simulink library "wt_blockset_beta"  (Simulink 5.0)
values from neighbouring files (symbols this model uses):
  a = -Le\Re    [matrix_coeff_trafo3limb_abc.m]
  a11 = K2*Rs/Ls    [matrix_coeff_scim_abc.m]    (also in matrix_coeff_spsm_dq.m = -Rs*Ksgm_frd/Ksgm_d; matrix_coeff_trafo_abc.m = K2*Rhv/Lhv; matrix_coeff_wrim_abc.m)
  a12 = K3*Rs/Ls    [matrix_coeff_scim_abc.m]    (also in matrix_coeff_spsm_dq.m = Lssq*Ksgm_frd/Ksgm_d; matrix_coeff_trafo_abc.m = K3*Rhv/Lhv; matrix_coeff_wrim_abc.m)
  a13 = 3*Msr*sqrt(3)*K4/4    [matrix_coeff_scim_abc.m]    (also in matrix_coeff_spsm_dq.m = Rf*Lsgm_rd*Lmd/Ksgm_d; matrix_coeff_trafo_abc.m = K4*Rhv; matrix_coeff_wrim_abc.m)
  a14 = K4*Rr    [matrix_coeff_scim_abc.m]    (also in matrix_coeff_spsm_dq.m = Rrd*Lsgm_f*Lmd/Ksgm_d; matrix_coeff_trafo_abc.m = K2/Lhv; matrix_coeff_wrim_abc.m)
  a15 = Msr*(K2-K3)/Ls    [matrix_coeff_scim_abc.m]    (also in matrix_coeff_spsm_dq.m = Lmq*Ksgm_frd/Ksgm_d; matrix_coeff_trafo_abc.m = K3/Lhv; matrix_coeff_wrim_abc.m)
  a16 = K2/Ls    [matrix_coeff_scim_abc.m]    (also in matrix_coeff_spsm_dq.m = Ksgm_frd/Ksgm_d; matrix_coeff_trafo_abc.m = K4; matrix_coeff_wrim_abc.m)
  a17 = K3/Ls    [matrix_coeff_scim_abc.m]    (also in matrix_coeff_spsm_dq.m = -Lsgm_rd*Lmd/Ksgm_d; matrix_coeff_wrim_abc.m)
  a21 = -Lssd*Lsrq/Ksgm_q    [matrix_coeff_spsm_dq.m]
  a22 = -Rs*Lsrq/Ksgm_q    [matrix_coeff_spsm_dq.m]
  a23 = -Lsrq*Lmd/Ksgm_q    [matrix_coeff_spsm_dq.m]
  a24 = -Lsrq*Lmd/Ksgm_q    [matrix_coeff_spsm_dq.m]
  a25 = Rrq*Lmq/Ksgm_q    [matrix_coeff_spsm_dq.m]
  a26 = Lsrq/Ksgm_q    [matrix_coeff_spsm_dq.m]
  a31 = K4*Rs    [matrix_coeff_scim_abc.m]    (also in matrix_coeff_spsm_dq.m = +Rs*Lsgm_rd*Lmd/Ksgm_d; matrix_coeff_trafo_abc.m = K4*Rlv; matrix_coeff_wrim_abc.m)
  a32 = Msr*(K2-K3)/Lr    [matrix_coeff_scim_abc.m]    (also in matrix_coeff_spsm_dq.m = -Lssq*Lsgm_rd*Lmd/Ksgm_d; matrix_coeff_trafo_abc.m = K2*Rlv/Llv; matrix_coeff_wrim_abc.m)
  a33 = K2*Rr/Lr    [matrix_coeff_scim_abc.m]    (also in matrix_coeff_spsm_dq.m = -Rf*Ksgm_srd/Ksgm_d; matrix_coeff_trafo_abc.m = K3*Rlv/Llv; matrix_coeff_wrim_abc.m)
  a34 = K3*Rr/Lr    [matrix_coeff_scim_abc.m]    (also in matrix_coeff_spsm_dq.m = Rrd*Lsgm_s*Lmd/Ksgm_d; matrix_coeff_trafo_abc.m = K4; matrix_coeff_wrim_abc.m)
  a35 = 3*Msr*sqrt(3)*K4/4    [matrix_coeff_scim_abc.m]    (also in matrix_coeff_spsm_dq.m = -Lsgm_rd*Lmd*Lmq/Ksgm_d; matrix_coeff_trafo_abc.m = K2/Llv; matrix_coeff_wrim_abc.m)
  a36 = K4    [matrix_coeff_scim_abc.m]    (also in matrix_coeff_spsm_dq.m = -Lsgm_rd*Lmd/Ksgm_d; matrix_coeff_trafo_abc.m = K3/Llv; matrix_coeff_wrim_abc.m)
  a37 = Ksgm_srd/Ksgm_d    [matrix_coeff_spsm_dq.m]    (also in matrix_coeff_wrim_abc.m = K2/Lr)
  a41 = Rs*Lsgm_f*Lmd/Ksgm_d    [matrix_coeff_spsm_dq.m]
  a42 = -Lsgm_f*Lssq*Lmd/Ksgm_d    [matrix_coeff_spsm_dq.m]
  a43 = Rf*Lsgm_s*Lmd/Ksgm_d    [matrix_coeff_spsm_dq.m]
  a44 = -Rrd*Ksgm_sf/Ksgm_d    [matrix_coeff_spsm_dq.m]
  a45 = -Lsgm_f*Lmd*Lmq/Ksgm_d    [matrix_coeff_spsm_dq.m]
  a46 = -Lsgm_f*Lmd/Ksgm_d    [matrix_coeff_spsm_dq.m]
  a47 = -Lsgm_s*Lmd/Ksgm_d    [matrix_coeff_spsm_dq.m]
  a51 = Lssd*Lmq/Ksgm_q    [matrix_coeff_spsm_dq.m]
  a52 = Rs*Lmq/Ksgm_q    [matrix_coeff_spsm_dq.m]
  a53 = Lmd*Lmq/Ksgm_q    [matrix_coeff_spsm_dq.m]
  a54 = Lmd*Lmq/Ksgm_q    [matrix_coeff_spsm_dq.m]
  a55 = -Rrq*Lssq/Ksgm_q    [matrix_coeff_spsm_dq.m]
  a56 = -Lmq/Ksgm_q    [matrix_coeff_spsm_dq.m]
  alpha_T = Ubase_hv/Ubase_lv    [matrix_coeff_trafo3limb_abc.m]
  b = inv(Le)    [matrix_coeff_trafo3limb_abc.m]
  Ctorque = cq(2:5:102,2:5:182)    [cq_table.m]
  Lmd = mag_ind(1)    [matrix_coeff_spsm_dq.m]
  Lmq = mag_ind(2)    [matrix_coeff_spsm_dq.m]
  Lss = Lsgms+Lm    [init_dbe_dq_scim.m]
  omg_base = 2*pi*rated_fp(1)    [init_dbe_dq_scim.m]    (also in init_dbe_rms_scim.m)
  p = rated_fp(2)    [init_dbe_dq_scim.m]    (also in init_dbe_rms_scim.m)
  Rs = stator(1)    [init_dbe_dq_scim.m]    (also in init_dbe_rms_scim.m; matrix_coeff_scim_abc.m; matrix_coeff_spsm_dq.m = stator_winding(1); matrix_coeff_wrim_abc.m)
  Xs = omg_base*Lss    [init_dbe_dq_scim.m]    (also in init_dbe_rms_scim.m = Xsgm_s+Xm)
undefined symbols (not defined in the file or in its folder): get, j, Kmode, ModeOp, Type, u0
libraries: simulink_extras x12, simulink x4, dspinverses x1, dspmtrx3 x1, dspsigattribs x1, dspspect3 x1
(part 4 of 4)

== system wt_blockset_beta/Mechanical Components/Wind Model SB-2/Kaimal_Filter_2/Kaimal Filter ==
  avg_wind : Inport
  In : Inport  Port=2
  A/D : Gain  Gain=0.0182/1.3463  SaturateOnIntegerOverflow=on
  Coefficients : Subsystem
  Integrator : Integrator  Orientation=up
  Integrator1 : Integrator  Orientation=up
  Product : Product  SaturateOnIntegerOverflow=on
  Product1 : Product  SaturateOnIntegerOverflow=on
  Product2 : Product  Orientation=left  SaturateOnIntegerOverflow=on
  Product3 : Product  Orientation=left  SaturateOnIntegerOverflow=on
  Sum : Sum  Inputs=|++  SaturateOnIntegerOverflow=on
  Sum1 : Sum  Orientation=up  Inputs=++-  SaturateOnIntegerOverflow=on
  Sum2 : Sum  Orientation=up  Inputs=+|-  SaturateOnIntegerOverflow=on
  Out : Outport
  wires:
  avg_wind/1 -> Coefficients/1(avg_wind)
  Coefficients/4(FD) -> [FD]
  Coefficients/3(ED) -> [ED]
  Coefficients/2(CD) -> [CD]
  Coefficients/1(BD) -> [BD]
  [FD] -> Product3/2
  [ED] -> Product2/2
  [CD] -> Product1/2
  [BD] -> Product/2
  In/1 -> Product1/1, Product/1, A/D/1
  Sum/1 -> Out/1, Product3/1, Product2/1
  Product1/1 -> Sum2/1
  Product3/1 -> Sum2/2
  Sum2/1 -> Integrator1/1
  Product2/1 -> Sum1/3
  Integrator1/1 -> Sum1/2
  Product/1 -> Sum1/1
  Sum1/1 -> Integrator/1
  Integrator/1 -> Sum/2
  A/D/1 -> Sum/1

== system wt_blockset_beta/Mechanical Components/Wind Model SB-2/Kaimal_Filter_3/Kaimal Filter ==
  avg_wind : Inport
  In : Inport  Port=2
  A/D : Gain  Gain=0.0182/1.3463  SaturateOnIntegerOverflow=on
  Coefficients : Subsystem
  Integrator : Integrator  Orientation=up
  Integrator1 : Integrator  Orientation=up
  Product : Product  SaturateOnIntegerOverflow=on
  Product1 : Product  SaturateOnIntegerOverflow=on
  Product2 : Product  Orientation=left  SaturateOnIntegerOverflow=on
  Product3 : Product  Orientation=left  SaturateOnIntegerOverflow=on
  Sum : Sum  Inputs=|++  SaturateOnIntegerOverflow=on
  Sum1 : Sum  Orientation=up  Inputs=++-  SaturateOnIntegerOverflow=on
  Sum2 : Sum  Orientation=up  Inputs=+|-  SaturateOnIntegerOverflow=on
  Out : Outport
  wires:
  A/D/1 -> Sum/1
  Integrator/1 -> Sum/2
  Sum1/1 -> Integrator/1
  Product/1 -> Sum1/1
  Integrator1/1 -> Sum1/2
  Product2/1 -> Sum1/3
  Sum2/1 -> Integrator1/1
  Product3/1 -> Sum2/2
  Product1/1 -> Sum2/1
  Sum/1 -> Product2/1, Product3/1, Out/1
  In/1 -> A/D/1, Product/1, Product1/1
  [BD] -> Product/2
  [CD] -> Product1/2
  [ED] -> Product2/2
  [FD] -> Product3/2
  Coefficients/1(BD) -> [BD]
  Coefficients/2(CD) -> [CD]
  Coefficients/3(ED) -> [ED]
  Coefficients/4(FD) -> [FD]
  avg_wind/1 -> Coefficients/1(avg_wind)

== system wt_blockset_beta/Mechanical Components/Wind Model SB-2/ZERO_Harmonic_Filter/ZERO harmonic Filter ==
  avg_wind : Inport
  In : Inport  Port=2
  Coefficients : Subsystem
  Integrator : Integrator  Orientation=up
  Integrator1 : Integrator  Orientation=up
  Product : Product  SaturateOnIntegerOverflow=on
  Product1 : Product  SaturateOnIntegerOverflow=on
  Product2 : Product  Orientation=left  SaturateOnIntegerOverflow=on
  Product3 : Product  Orientation=left  SaturateOnIntegerOverflow=on
  Sum1 : Sum  Orientation=up  Inputs=++-  SaturateOnIntegerOverflow=on
  Sum2 : Sum  Orientation=up  Inputs=+|-  SaturateOnIntegerOverflow=on
  Out : Outport
  wires:
  avg_wind/1 -> Coefficients/1(avg_wind)
  Coefficients/4(FD) -> [FD]
  Coefficients/3(ED) -> [ED]
  Coefficients/2(CD) -> [CD]
  Coefficients/1(BD) -> [BD]
  [FD] -> Product3/2
  [ED] -> Product2/2
  [CD] -> Product1/2
  [BD] -> Product/2
  In/1 -> Product1/1, Product/1
  Product1/1 -> Sum2/1
  Product3/1 -> Sum2/2
  Sum2/1 -> Integrator1/1
  Product2/1 -> Sum1/3
  Integrator1/1 -> Sum1/2
  Product/1 -> Sum1/1
  Sum1/1 -> Integrator/1
  Integrator/1 -> Out/1, Product3/1, Product2/1

== system wt_blockset_beta/Power Converters/3-phase Diode Bridge Rectifier/Diode  State Calculator/Branch A+ ==
  RST : Inport
  Demux2 : Demux  Outputs=3
  Logical Operator : Logic
  Relational Operator : RelationalOperator  InputSameDT=on
  Relational Operator1 : RelationalOperator  Operator=>  InputSameDT=on
  A : Outport  InitialOutput=0
  wires:
  Relational Operator/1 -> Logical Operator/1
  Relational Operator1/1 -> Logical Operator/2
  Logical Operator/1 -> A/1
  RST/1 -> Demux2/1
  Demux2/1 -> Relational Operator/1, Relational Operator1/1
  Demux2/3 -> Relational Operator/2
  Demux2/2 -> Relational Operator1/2

== system wt_blockset_beta/Power Converters/3-phase Diode Bridge Rectifier/Diode  State Calculator/Branch A- ==
  RST : Inport
  Demux2 : Demux  Outputs=3
  Logical Operator : Logic
  Relational Operator : RelationalOperator  Operator=<  InputSameDT=on
  Relational Operator1 : RelationalOperator  Operator=<  InputSameDT=on
  A : Outport  InitialOutput=0
  wires:
  Demux2/2 -> Relational Operator1/2
  Demux2/3 -> Relational Operator/2
  Demux2/1 -> Relational Operator1/1, Relational Operator/1
  RST/1 -> Demux2/1
  Logical Operator/1 -> A/1
  Relational Operator1/1 -> Logical Operator/2
  Relational Operator/1 -> Logical Operator/1

== system wt_blockset_beta/Power Converters/3-phase Diode Bridge Rectifier/Diode  State Calculator/Branch B+ ==
  RST : Inport
  Demux2 : Demux  Outputs=3
  Logical Operator : Logic
  Relational Operator : RelationalOperator  InputSameDT=on
  Relational Operator1 : RelationalOperator  Operator=>  InputSameDT=on
  B : Outport  InitialOutput=0
  wires:
  RST/1 -> Demux2/1
  Logical Operator/1 -> B/1
  Relational Operator1/1 -> Logical Operator/2
  Relational Operator/1 -> Logical Operator/1
  Demux2/2 -> Relational Operator/1, Relational Operator1/1
  Demux2/1 -> Relational Operator/2
  Demux2/3 -> Relational Operator1/2

== system wt_blockset_beta/Power Converters/3-phase Diode Bridge Rectifier/Diode  State Calculator/Branch B- ==
  RST : Inport
  Demux2 : Demux  Outputs=3
  Logical Operator : Logic
  Relational Operator : RelationalOperator  Operator=<  InputSameDT=on
  Relational Operator1 : RelationalOperator  Operator=<  InputSameDT=on
  B : Outport  InitialOutput=0
  wires:
  Demux2/3 -> Relational Operator1/2
  Demux2/1 -> Relational Operator/2
  Demux2/2 -> Relational Operator1/1, Relational Operator/1
  Relational Operator/1 -> Logical Operator/1
  Relational Operator1/1 -> Logical Operator/2
  Logical Operator/1 -> B/1
  RST/1 -> Demux2/1

== system wt_blockset_beta/Power Converters/3-phase Diode Bridge Rectifier/Diode  State Calculator/Branch C+ ==
  RST : Inport
  Demux2 : Demux  Outputs=3
  Logical Operator : Logic
  Relational Operator : RelationalOperator  InputSameDT=on
  Relational Operator1 : RelationalOperator  Operator=>  InputSameDT=on
  C : Outport  InitialOutput=0
  wires:
  Relational Operator/1 -> Logical Operator/1
  Relational Operator1/1 -> Logical Operator/2
  Logical Operator/1 -> C/1
  RST/1 -> Demux2/1
  Demux2/3 -> Relational Operator/1, Relational Operator1/1
  Demux2/2 -> Relational Operator/2
  Demux2/1 -> Relational Operator1/2

== system wt_blockset_beta/Power Converters/3-phase Diode Bridge Rectifier/Diode  State Calculator/Branch C- ==
  RST : Inport
  Demux2 : Demux  Outputs=3
  Logical Operator : Logic
  Relational Operator : RelationalOperator  Operator=<  InputSameDT=on
  Relational Operator1 : RelationalOperator  Operator=<  InputSameDT=on
  C : Outport  InitialOutput=0
  wires:
  Demux2/1 -> Relational Operator1/2
  Demux2/2 -> Relational Operator/2
  Demux2/3 -> Relational Operator1/1, Relational Operator/1
  RST/1 -> Demux2/1
  Logical Operator/1 -> C/1
  Relational Operator1/1 -> Logical Operator/2
  Relational Operator/1 -> Logical Operator/1

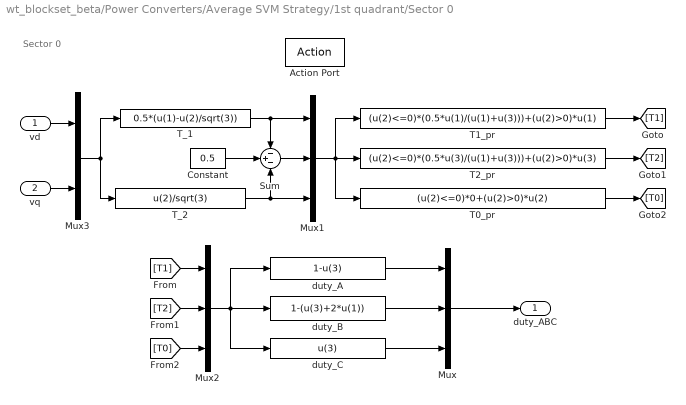
== system wt_blockset_beta/Power Converters/Average SVM Strategy/1st quadrant/Sector 0 ==
  note: Sector 0
  vd : Inport
  vq : Inport  Port=2
  Action Port : ActionPort  InitializeStates=reset
  Constant : Constant  Value=0.5
  Mux : Mux  Inputs=3
  Mux1 : Mux  Inputs=3
  Mux2 : Mux  Inputs=3
  Mux3 : Mux  Inputs=2
  Sum : Sum  Inputs=-+-  SaturateOnIntegerOverflow=on
  T0_pr : Fcn  Expr=(u(2)<=0)*0+(u(2)>0)*u(2)
  T1_pr : Fcn  Expr=(u(2)<=0)*(0.5*u(1)/(u(1)+u(3)))+(u(2)>0)*u(1)
  T2_pr : Fcn  Expr=(u(2)<=0)*(0.5*u(3)/(u(1)+u(3)))+(u(2)>0)*u(3)
  T_1 : Fcn  Expr=0.5*(u(1)-u(2)/sqrt(3))
  T_2 : Fcn  Expr=u(2)/sqrt(3)
  duty_A : Fcn  Expr=1-u(3)
  duty_B : Fcn  Expr=1-(u(3)+2*u(1))
  duty_C : Fcn  Expr=u(3)
  duty_ABC : Outport  OutputWhenDisabled=reset  InitialOutput=[0 0 0]
  wires:
  T_2/1 -> Sum/3, Mux1/3
  T_1/1 -> Sum/1, Mux1/1
  Constant/1 -> Sum/2
  Sum/1 -> Mux1/2
  T1_pr/1 -> [T1]
  T2_pr/1 -> [T2]
  T0_pr/1 -> [T0]
  Mux1/1 -> T1_pr/1, T2_pr/1, T0_pr/1
  [T1] -> Mux2/1
  [T2] -> Mux2/2
  [T0] -> Mux2/3
  Mux2/1 -> duty_B/1, duty_A/1, duty_C/1
  duty_A/1 -> Mux/1
  duty_B/1 -> Mux/2
  duty_C/1 -> Mux/3
  Mux/1 -> duty_ABC/1
  Mux3/1 -> T_1/1, T_2/1
  vd/1 -> Mux3/1
  vq/1 -> Mux3/2

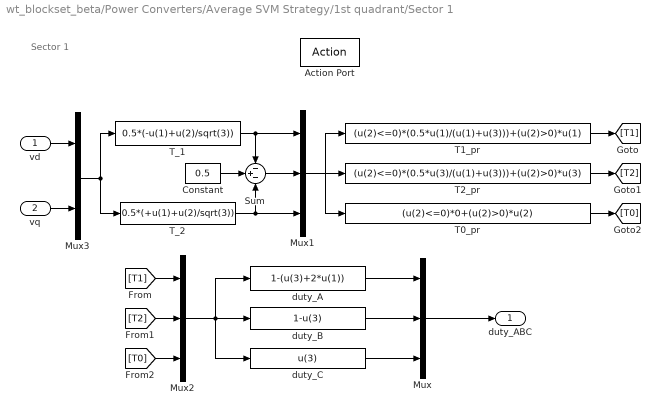
== system wt_blockset_beta/Power Converters/Average SVM Strategy/1st quadrant/Sector 1 ==
  note: Sector 1
  vd : Inport
  vq : Inport  Port=2
  Action Port : ActionPort  InitializeStates=reset
  Constant : Constant  Value=0.5
  Mux : Mux  Inputs=3
  Mux1 : Mux  Inputs=3
  Mux2 : Mux  Inputs=3
  Mux3 : Mux  Inputs=2
  Sum : Sum  Inputs=-+-  SaturateOnIntegerOverflow=on
  T0_pr : Fcn  Expr=(u(2)<=0)*0+(u(2)>0)*u(2)
  T1_pr : Fcn  Expr=(u(2)<=0)*(0.5*u(1)/(u(1)+u(3)))+(u(2)>0)*u(1)
  T2_pr : Fcn  Expr=(u(2)<=0)*(0.5*u(3)/(u(1)+u(3)))+(u(2)>0)*u(3)
  T_1 : Fcn  Expr=0.5*(-u(1)+u(2)/sqrt(3))
  T_2 : Fcn  Expr=0.5*(+u(1)+u(2)/sqrt(3))
  duty_A : Fcn  Expr=1-(u(3)+2*u(1))
  duty_B : Fcn  Expr=1-u(3)
  duty_C : Fcn  Expr=u(3)
  duty_ABC : Outport  OutputWhenDisabled=reset  InitialOutput=[0 0 0]
  wires:
  Sum/1 -> Mux1/2
  Constant/1 -> Sum/2
  T_1/1 -> Sum/1, Mux1/1
  T_2/1 -> Mux1/3, Sum/3
  Mux1/1 -> T1_pr/1, T2_pr/1, T0_pr/1
  T1_pr/1 -> [T1]
  T2_pr/1 -> [T2]
  T0_pr/1 -> [T0]
  [T1] -> Mux2/1
  [T2] -> Mux2/2
  [T0] -> Mux2/3
  Mux/1 -> duty_ABC/1
  Mux2/1 -> duty_B/1, duty_A/1, duty_C/1
  duty_B/1 -> Mux/2
  duty_A/1 -> Mux/1
  duty_C/1 -> Mux/3
  Mux3/1 -> T_1/1, T_2/1
  vq/1 -> Mux3/2
  vd/1 -> Mux3/1

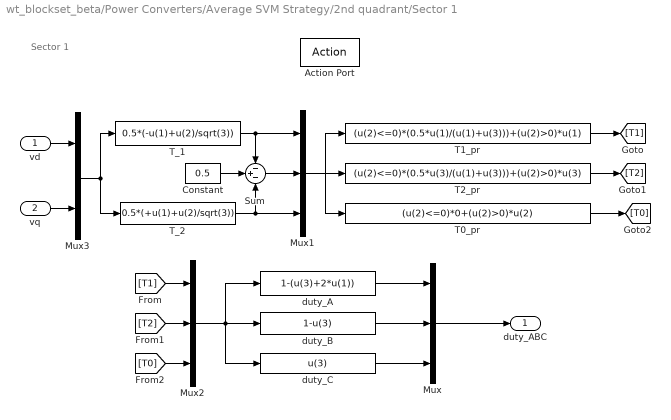
== system wt_blockset_beta/Power Converters/Average SVM Strategy/2nd quadrant/Sector 1 ==
  note: Sector 1
  vd : Inport
  vq : Inport  Port=2
  Action Port : ActionPort  InitializeStates=reset
  Constant : Constant  Value=0.5
  Mux : Mux  Inputs=3
  Mux1 : Mux  Inputs=3
  Mux2 : Mux  Inputs=3
  Mux3 : Mux  Inputs=2
  Sum : Sum  Inputs=-+-  SaturateOnIntegerOverflow=on
  T0_pr : Fcn  Expr=(u(2)<=0)*0+(u(2)>0)*u(2)
  T1_pr : Fcn  Expr=(u(2)<=0)*(0.5*u(1)/(u(1)+u(3)))+(u(2)>0)*u(1)
  T2_pr : Fcn  Expr=(u(2)<=0)*(0.5*u(3)/(u(1)+u(3)))+(u(2)>0)*u(3)
  T_1 : Fcn  Expr=0.5*(-u(1)+u(2)/sqrt(3))
  T_2 : Fcn  Expr=0.5*(+u(1)+u(2)/sqrt(3))
  duty_A : Fcn  Expr=1-(u(3)+2*u(1))
  duty_B : Fcn  Expr=1-u(3)
  duty_C : Fcn  Expr=u(3)
  duty_ABC : Outport  OutputWhenDisabled=reset  InitialOutput=[0 0 0]
  wires:
  Sum/1 -> Mux1/2
  Constant/1 -> Sum/2
  T_1/1 -> Sum/1, Mux1/1
  T_2/1 -> Mux1/3, Sum/3
  Mux1/1 -> T1_pr/1, T2_pr/1, T0_pr/1
  T1_pr/1 -> [T1]
  T2_pr/1 -> [T2]
  T0_pr/1 -> [T0]
  [T1] -> Mux2/1
  [T2] -> Mux2/2
  [T0] -> Mux2/3
  Mux/1 -> duty_ABC/1
  Mux2/1 -> duty_B/1, duty_A/1, duty_C/1
  duty_B/1 -> Mux/2
  duty_A/1 -> Mux/1
  duty_C/1 -> Mux/3
  Mux3/1 -> T_1/1, T_2/1
  vq/1 -> Mux3/2
  vd/1 -> Mux3/1

== system wt_blockset_beta/Power Converters/Average SVM Strategy/2nd quadrant/Sector 2 ==
  note: Sector 2
  vd : Inport
  vq : Inport  Port=2
  Action Port : ActionPort  InitializeStates=reset
  Constant : Constant  Value=0.5
  Mux : Mux  Inputs=3
  Mux1 : Mux  Inputs=3
  Mux2 : Mux  Inputs=3
  Mux3 : Mux  Inputs=2
  Sum : Sum  Inputs=-+-  SaturateOnIntegerOverflow=on
  T0_pr : Fcn  Expr=(u(2)<=0)*0+(u(2)>0)*u(2)
  T1_pr : Fcn  Expr=(u(2)<=0)*(0.5*u(1)/(u(1)+u(3)))+(u(2)>0)*u(1)
  T2_pr : Fcn  Expr=(u(2)<=0)*(0.5*u(3)/(u(1)+u(3)))+(u(2)>0)*u(3)
  T_ : Fcn  Expr=0.5*(abs(u(1))-u(2)/sqrt(3))
  T_1 : Fcn  Expr=u(2)/sqrt(3)
  duty_A : Fcn  Expr=u(3)
  duty_B : Fcn  Expr=1-u(3)
  duty_C : Fcn  Expr=1-(u(3)+2*u(1))
  duty_ABC : Outport  OutputWhenDisabled=reset  InitialOutput=[0 0 0]
  wires:
  Mux/1 -> duty_ABC/1
  [T0] -> Mux2/3
  [T2] -> Mux2/2
  [T1] -> Mux2/1
  Mux1/1 -> T0_pr/1, T2_pr/1, T1_pr/1
  T0_pr/1 -> [T0]
  T2_pr/1 -> [T2]
  T1_pr/1 -> [T1]
  Sum/1 -> Mux1/2
  Constant/1 -> Sum/2
  vq/1 -> Mux3/2
  vd/1 -> Mux3/1
  Mux3/1 -> T_1/1, T_/1
  T_1/1 -> Mux1/1, Sum/1
  T_/1 -> Mux1/3, Sum/3
  duty_B/1 -> Mux/2
  duty_A/1 -> Mux/1
  duty_C/1 -> Mux/3
  Mux2/1 -> duty_B/1, duty_A/1, duty_C/1

== system wt_blockset_beta/Power Converters/Average SVM Strategy/3rd quadrant/Sector 3 ==
  note: Sector 2
  vd : Inport
  vq : Inport  Port=2
  Action Port : ActionPort  InitializeStates=reset
  Constant : Constant  Value=0.5
  Mux : Mux  Inputs=3
  Mux1 : Mux  Inputs=3
  Mux2 : Mux  Inputs=3
  Mux3 : Mux  Inputs=2
  Sum : Sum  Inputs=-+-  SaturateOnIntegerOverflow=on
  T0_pr : Fcn  Expr=(u(2)<=0)*0+(u(2)>0)*u(2)
  T1_pr : Fcn  Expr=(u(2)<=0)*(0.5*u(1)/(u(1)+u(3)))+(u(2)>0)*u(1)
  T2_pr : Fcn  Expr=(u(2)<=0)*(0.5*u(3)/(u(1)+u(3)))+(u(2)>0)*u(3)
  T_ : Fcn  Expr=0.5*(abs(u(1))-abs(u(2))/sqrt(3))
  T_1 : Fcn  Expr=abs(u(2))/sqrt(3)
  duty_A : Fcn  Expr=u(3)
  duty_B : Fcn  Expr=1-(u(3)+2*u(1))
  duty_C : Fcn  Expr=1-u(3)
  duty_ABC : Outport  OutputWhenDisabled=reset  InitialOutput=[0 0 0]
  wires:
  Mux/1 -> duty_ABC/1
  [T0] -> Mux2/3
  [T2] -> Mux2/2
  [T1] -> Mux2/1
  Mux1/1 -> T0_pr/1, T2_pr/1, T1_pr/1
  T0_pr/1 -> [T0]
  T2_pr/1 -> [T2]
  T1_pr/1 -> [T1]
  Sum/1 -> Mux1/2
  Constant/1 -> Sum/2
  vq/1 -> Mux3/2
  vd/1 -> Mux3/1
  Mux3/1 -> T_1/1, T_/1
  T_1/1 -> Mux1/1, Sum/1
  T_/1 -> Mux1/3, Sum/3
  duty_A/1 -> Mux/1
  Mux2/1 -> duty_A/1, duty_B/1, duty_C/1
  duty_B/1 -> Mux/2
  duty_C/1 -> Mux/3

== system wt_blockset_beta/Power Converters/Average SVM Strategy/3rd quadrant/Sector 4 ==
  note: Sector 4
  vd : Inport
  vq : Inport  Port=2
  Action Port : ActionPort  InitializeStates=reset
  Constant : Constant  Value=0.5
  Mux : Mux  Inputs=3
  Mux1 : Mux  Inputs=3
  Mux2 : Mux  Inputs=3
  Mux3 : Mux  Inputs=2
  Sum : Sum  Inputs=-+-  SaturateOnIntegerOverflow=on
  T0_pr : Fcn  Expr=(u(2)<=0)*0+(u(2)>0)*u(2)
  T1_pr : Fcn  Expr=(u(2)<=0)*(0.5*u(1)/(u(1)+u(3)))+(u(2)>0)*u(1)
  T2_pr : Fcn  Expr=(u(2)<=0)*(0.5*u(3)/(u(1)+u(3)))+(u(2)>0)*u(3)
  T_1 : Fcn  Expr=0.5*(-u(1)+abs(u(2))/sqrt(3))
  T_2 : Fcn  Expr=0.5*(u(1)+abs(u(2))/sqrt(3))
  duty_A : Fcn  Expr=1-(u(3)+2*u(1))
  duty_B : Fcn  Expr=u(3)
  duty_C : Fcn  Expr=1-u(3)
  duty_ABC : Outport  OutputWhenDisabled=reset  InitialOutput=[0 0 0]
  wires:
  Sum/1 -> Mux1/2
  Constant/1 -> Sum/2
  T_1/1 -> Sum/1, Mux1/1
  T_2/1 -> Mux1/3, Sum/3
  Mux1/1 -> T1_pr/1, T2_pr/1, T0_pr/1
  T0_pr/1 -> [T0]
  T1_pr/1 -> [T1]
  T2_pr/1 -> [T2]
  [T1] -> Mux2/1
  [T2] -> Mux2/2
  [T0] -> Mux2/3
  Mux/1 -> duty_ABC/1
  Mux2/1 -> duty_A/1, duty_B/1, duty_C/1
  duty_A/1 -> Mux/1
  Mux3/1 -> T_1/1, T_2/1
  vq/1 -> Mux3/2
  vd/1 -> Mux3/1
  duty_B/1 -> Mux/2
  duty_C/1 -> Mux/3

== system wt_blockset_beta/Power Converters/Average SVM Strategy/4th quadrant/Sector 4 ==
  note: Sector 4
  vd : Inport
  vq : Inport  Port=2
  Action Port : ActionPort  InitializeStates=reset
  Constant : Constant  Value=0.5
  Mux : Mux  Inputs=3
  Mux1 : Mux  Inputs=3
  Mux2 : Mux  Inputs=3
  Mux3 : Mux  Inputs=2
  Sum : Sum  Inputs=-+-  SaturateOnIntegerOverflow=on
  T0_pr : Fcn  Expr=(u(2)<=0)*0+(u(2)>0)*u(2)
  T1_pr : Fcn  Expr=(u(2)<=0)*(0.5*u(1)/(u(1)+u(3)))+(u(2)>0)*u(1)
  T2_pr : Fcn  Expr=(u(2)<=0)*(0.5*u(3)/(u(1)+u(3)))+(u(2)>0)*u(3)
  T_1 : Fcn  Expr=0.5*(-u(1)+abs(u(2))/sqrt(3))
  T_2 : Fcn  Expr=0.5*(u(1)+abs(u(2))/sqrt(3))
  duty_A : Fcn  Expr=1-(u(3)+2*u(1))
  duty_B : Fcn  Expr=u(3)
  duty_C : Fcn  Expr=1-u(3)
  duty_ABC : Outport  OutputWhenDisabled=reset  InitialOutput=[0 0 0]
  wires:
  duty_C/1 -> Mux/3
  duty_B/1 -> Mux/2
  vd/1 -> Mux3/1
  vq/1 -> Mux3/2
  Mux3/1 -> T_2/1, T_1/1
  duty_A/1 -> Mux/1
  Mux2/1 -> duty_C/1, duty_B/1, duty_A/1
  Mux/1 -> duty_ABC/1
  [T0] -> Mux2/3
  [T2] -> Mux2/2
  [T1] -> Mux2/1
  T0_pr/1 -> [T0]
  T2_pr/1 -> [T2]
  T1_pr/1 -> [T1]
  Mux1/1 -> T0_pr/1, T2_pr/1, T1_pr/1
  T_2/1 -> Sum/3, Mux1/3
  T_1/1 -> Mux1/1, Sum/1
  Constant/1 -> Sum/2
  Sum/1 -> Mux1/2

== system wt_blockset_beta/Power Converters/Average SVM Strategy/4th quadrant/Sector 5 ==
  note: Sector 5
  vd : Inport
  vq : Inport  Port=2
  Action Port : ActionPort  InitializeStates=reset
  Constant : Constant  Value=0.5
  Mux : Mux  Inputs=3
  Mux1 : Mux  Inputs=3
  Mux2 : Mux  Inputs=3
  Mux3 : Mux  Inputs=2
  Sum : Sum  Inputs=-+-  SaturateOnIntegerOverflow=on
  T0_pr : Fcn  Expr=(u(2)<=0)*0+(u(2)>0)*u(2)
  T1_pr : Fcn  Expr=(u(2)<=0)*(0.5*u(1)/(u(1)+u(3)))+(u(2)>0)*u(1)
  T2_pr : Fcn  Expr=(u(2)<=0)*(0.5*u(3)/(u(1)+u(3)))+(u(2)>0)*u(3)
  T_1 : Fcn  Expr=0.5*((u(1))-abs(u(2))/sqrt(3))
  T_2 : Fcn  Expr=abs(u(2))/sqrt(3)
  duty_A : Fcn  Expr=1-u(3)
  duty_B : Fcn  Expr=u(3)
  duty_C : Fcn  Expr=1-(u(3)+2*u(1))
  duty_ABC : Outport  OutputWhenDisabled=reset  InitialOutput=[0 0 0]
  wires:
  vd/1 -> Mux3/1
  vq/1 -> Mux3/2
  Constant/1 -> Sum/2
  Sum/1 -> Mux1/2
  T1_pr/1 -> [T1]
  T2_pr/1 -> [T2]
  T0_pr/1 -> [T0]
  Mux1/1 -> T1_pr/1, T2_pr/1, T0_pr/1
  [T1] -> Mux2/1
  [T2] -> Mux2/2
  [T0] -> Mux2/3
  Mux/1 -> duty_ABC/1
  T_2/1 -> Mux1/3, Sum/3
  T_1/1 -> Mux1/1, Sum/1
  Mux3/1 -> T_1/1, T_2/1
  duty_A/1 -> Mux/1
  duty_B/1 -> Mux/2
  duty_C/1 -> Mux/3
  Mux2/1 -> duty_B/1, duty_A/1, duty_C/1

== system wt_blockset_beta/Power Converters/Switching PWM Strategy/capcom/Vtri1 ==
  Constant1 : Constant
  Constant2 : Constant
  Constant3 : Constant  Value=0
  Data Type Conversion : DataTypeConversion  SaturateOnIntegerOverflow=on
  Fcn : Fcn  Expr=-u(1)*2+1
  Gain : Gain  Gain=fsw2  SaturateOnIntegerOverflow=on
  Gain1 : Gain  Gain=2*fsw2  SaturateOnIntegerOverflow=on
  IC : InitialCondition  Value=1.5
  Integrator : Integrator  ExternalReset=rising  InitialConditionSource=external  InitialCondition=1.5
  Integrator1 : Integrator  ExternalReset=rising
  Pulse Generator : DiscretePulseGenerator  PulseType=Time based  Period=2/fsw2  PulseWidth=50  PhaseDelay=0.5/fsw2
  Pulse Generator1 : DiscretePulseGenerator  PulseType=Time based  Period=2/fsw2  PulseWidth=50
  Relational Operator : RelationalOperator  InputSameDT=on
  Vtri : Outport  InitialOutput=0
  wires:
  Integrator1/1 -> Vtri/1
  Pulse Generator/1 -> Integrator/2
  Constant2/1 -> Gain/1
  Fcn/1 -> Gain1/1
  Relational Operator/1 -> Data Type Conversion/1
  Integrator/1 -> Relational Operator/1
  IC/1 -> Integrator/3
  Constant3/1 -> IC/1
  Pulse Generator1/1 -> Integrator1/2
  Gain1/1 -> Integrator1/1
  Gain/1 -> Integrator/1
  Constant1/1 -> Relational Operator/2
  Data Type Conversion/1 -> Fcn/1

== system wt_blockset_beta/Power Converters/Switching PWM Strategy/capcom/pulses ==
  In1 : Inport
  Constant : Constant  Value=0
  Data Type Conversion : DataTypeConversion  DataType=double  SaturateOnIntegerOverflow=on
  Hit  Crossing : HitCross  ShowOutputPort=off
  IC : InitialCondition  Value=0
  Relational Operator : RelationalOperator  InputSameDT=on
  Out1 : Outport  InitialOutput=0
  wires:
  Relational Operator/1 -> Data Type Conversion/1
  In1/1 -> Relational Operator/1
  Constant/1 -> Relational Operator/2
  IC/1 -> Out1/1
  Data Type Conversion/1 -> Hit  Crossing/1, IC/1

== system wt_blockset_beta/Power Converters/Switching SVM Strategy/1st quadrant/Sector 0 ==
  note: Sector 0
  vd : Inport
  vq : Inport  Port=2
  Action Port : ActionPort  InitializeStates=reset
  Constant : Constant  Value=0.5
  Mux : Mux  Inputs=3
  Mux1 : Mux  Inputs=3
  Mux2 : Mux  Inputs=3
  Mux3 : Mux  Inputs=2
  Sum : Sum  Inputs=-+-  SaturateOnIntegerOverflow=on
  T0_pr : Fcn  Expr=(u(2)<=0)*0+(u(2)>0)*u(2)
  T1_pr : Fcn  Expr=(u(2)<=0)*(0.5*u(1)/(u(1)+u(3)))+(u(2)>0)*u(1)
  T2_pr : Fcn  Expr=(u(2)<=0)*(0.5*u(3)/(u(1)+u(3)))+(u(2)>0)*u(3)
  T_1 : Fcn  Expr=0.5*(u(1)-u(2)/sqrt(3))
  T_2 : Fcn  Expr=u(2)/sqrt(3)
  duty_A : Fcn  Expr=1-u(3)
  duty_B : Fcn  Expr=1-(u(3)+2*u(1))
  duty_C : Fcn  Expr=u(3)
  duty_ABC : Outport  OutputWhenDisabled=reset  InitialOutput=[0 0 0]
  wires:
  T_2/1 -> Sum/3, Mux1/3
  T_1/1 -> Sum/1, Mux1/1
  Constant/1 -> Sum/2
  Sum/1 -> Mux1/2
  T1_pr/1 -> [T1]
  T2_pr/1 -> [T2]
  T0_pr/1 -> [T0]
  Mux1/1 -> T1_pr/1, T2_pr/1, T0_pr/1
  [T1] -> Mux2/1
  [T2] -> Mux2/2
  [T0] -> Mux2/3
  Mux2/1 -> duty_B/1, duty_A/1, duty_C/1
  duty_A/1 -> Mux/1
  duty_B/1 -> Mux/2
  duty_C/1 -> Mux/3
  Mux/1 -> duty_ABC/1
  Mux3/1 -> T_1/1, T_2/1
  vd/1 -> Mux3/1
  vq/1 -> Mux3/2

== system wt_blockset_beta/Power Converters/Switching SVM Strategy/1st quadrant/Sector 1 ==
  note: Sector 1
  vd : Inport
  vq : Inport  Port=2
  Action Port : ActionPort  InitializeStates=reset
  Constant : Constant  Value=0.5
  Mux : Mux  Inputs=3
  Mux1 : Mux  Inputs=3
  Mux2 : Mux  Inputs=3
  Mux3 : Mux  Inputs=2
  Sum : Sum  Inputs=-+-  SaturateOnIntegerOverflow=on
  T0_pr : Fcn  Expr=(u(2)<=0)*0+(u(2)>0)*u(2)
  T1_pr : Fcn  Expr=(u(2)<=0)*(0.5*u(1)/(u(1)+u(3)))+(u(2)>0)*u(1)
  T2_pr : Fcn  Expr=(u(2)<=0)*(0.5*u(3)/(u(1)+u(3)))+(u(2)>0)*u(3)
  T_1 : Fcn  Expr=0.5*(-u(1)+u(2)/sqrt(3))
  T_2 : Fcn  Expr=0.5*(+u(1)+u(2)/sqrt(3))
  duty_A : Fcn  Expr=1-(u(3)+2*u(1))
  duty_B : Fcn  Expr=1-u(3)
  duty_C : Fcn  Expr=u(3)
  duty_ABC : Outport  OutputWhenDisabled=reset  InitialOutput=[0 0 0]
  wires:
  Sum/1 -> Mux1/2
  Constant/1 -> Sum/2
  T_1/1 -> Sum/1, Mux1/1
  T_2/1 -> Mux1/3, Sum/3
  Mux1/1 -> T1_pr/1, T2_pr/1, T0_pr/1
  [T1] -> Mux2/1
  [T2] -> Mux2/2
  [T0] -> Mux2/3
  Mux/1 -> duty_ABC/1
  Mux2/1 -> duty_B/1, duty_A/1, duty_C/1
  duty_B/1 -> Mux/2
  duty_A/1 -> Mux/1
  duty_C/1 -> Mux/3
  Mux3/1 -> T_1/1, T_2/1
  vq/1 -> Mux3/2
  vd/1 -> Mux3/1
  T1_pr/1 -> [T1]
  T2_pr/1 -> [T2]
  T0_pr/1 -> [T0]

== system wt_blockset_beta/Power Converters/Switching SVM Strategy/2nd quadrant/Sector 1 ==
  note: Sector 1
  vd : Inport
  vq : Inport  Port=2
  Action Port : ActionPort  InitializeStates=reset
  Constant : Constant  Value=0.5
  Mux : Mux  Inputs=3
  Mux1 : Mux  Inputs=3
  Mux2 : Mux  Inputs=3
  Mux3 : Mux  Inputs=2
  Sum : Sum  Inputs=-+-  SaturateOnIntegerOverflow=on
  T0_pr : Fcn  Expr=(u(2)<=0)*0+(u(2)>0)*u(2)
  T1_pr : Fcn  Expr=(u(2)<=0)*(0.5*u(1)/(u(1)+u(3)))+(u(2)>0)*u(1)
  T2_pr : Fcn  Expr=(u(2)<=0)*(0.5*u(3)/(u(1)+u(3)))+(u(2)>0)*u(3)
  T_1 : Fcn  Expr=0.5*(-u(1)+u(2)/sqrt(3))
  T_2 : Fcn  Expr=0.5*(+u(1)+u(2)/sqrt(3))
  duty_A : Fcn  Expr=1-(u(3)+2*u(1))
  duty_B : Fcn  Expr=1-u(3)
  duty_C : Fcn  Expr=u(3)
  duty_ABC : Outport  OutputWhenDisabled=reset  InitialOutput=[0 0 0]
  wires:
  Sum/1 -> Mux1/2
  Constant/1 -> Sum/2
  T_1/1 -> Sum/1, Mux1/1
  T_2/1 -> Mux1/3, Sum/3
  Mux1/1 -> T1_pr/1, T2_pr/1, T0_pr/1
  [T1] -> Mux2/1
  [T2] -> Mux2/2
  [T0] -> Mux2/3
  Mux/1 -> duty_ABC/1
  Mux2/1 -> duty_B/1, duty_A/1, duty_C/1
  duty_B/1 -> Mux/2
  duty_A/1 -> Mux/1
  duty_C/1 -> Mux/3
  Mux3/1 -> T_1/1, T_2/1
  vq/1 -> Mux3/2
  vd/1 -> Mux3/1
  T1_pr/1 -> [T1]
  T2_pr/1 -> [T2]
  T0_pr/1 -> [T0]

== system wt_blockset_beta/Power Converters/Switching SVM Strategy/2nd quadrant/Sector 2 ==
  note: Sector 2
  vd : Inport
  vq : Inport  Port=2
  Action Port : ActionPort  InitializeStates=reset
  Constant : Constant  Value=0.5
  Mux : Mux  Inputs=3
  Mux1 : Mux  Inputs=3
  Mux2 : Mux  Inputs=3
  Mux3 : Mux  Inputs=2
  Sum : Sum  Inputs=-+-  SaturateOnIntegerOverflow=on
  T0_pr : Fcn  Expr=(u(2)<=0)*0+(u(2)>0)*u(2)
  T1_pr : Fcn  Expr=(u(2)<=0)*(0.5*u(1)/(u(1)+u(3)))+(u(2)>0)*u(1)
  T2_pr : Fcn  Expr=(u(2)<=0)*(0.5*u(3)/(u(1)+u(3)))+(u(2)>0)*u(3)
  T_ : Fcn  Expr=0.5*(abs(u(1))-u(2)/sqrt(3))
  T_1 : Fcn  Expr=u(2)/sqrt(3)
  duty_A : Fcn  Expr=u(3)
  duty_B : Fcn  Expr=1-u(3)
  duty_C : Fcn  Expr=1-(u(3)+2*u(1))
  duty_ABC : Outport  OutputWhenDisabled=reset  InitialOutput=[0 0 0]
  wires:
  Mux/1 -> duty_ABC/1
  [T0] -> Mux2/3
  [T2] -> Mux2/2
  [T1] -> Mux2/1
  Mux1/1 -> T0_pr/1, T2_pr/1, T1_pr/1
  Sum/1 -> Mux1/2
  Constant/1 -> Sum/2
  vq/1 -> Mux3/2
  vd/1 -> Mux3/1
  Mux3/1 -> T_1/1, T_/1
  T_1/1 -> Mux1/1, Sum/1
  T_/1 -> Mux1/3, Sum/3
  duty_B/1 -> Mux/2
  duty_A/1 -> Mux/1
  duty_C/1 -> Mux/3
  Mux2/1 -> duty_B/1, duty_A/1, duty_C/1
  T1_pr/1 -> [T1]
  T2_pr/1 -> [T2]
  T0_pr/1 -> [T0]

== system wt_blockset_beta/Power Converters/Switching SVM Strategy/3rd quadrant/Sector 3 ==
  note: Sector 2
  vd : Inport
  vq : Inport  Port=2
  Action Port : ActionPort  InitializeStates=reset
  Constant : Constant  Value=0.5
  Mux : Mux  Inputs=3
  Mux1 : Mux  Inputs=3
  Mux2 : Mux  Inputs=3
  Mux3 : Mux  Inputs=2
  Sum : Sum  Inputs=-+-  SaturateOnIntegerOverflow=on
  T0_pr : Fcn  Expr=(u(2)<=0)*0+(u(2)>0)*u(2)
  T1_pr : Fcn  Expr=(u(2)<=0)*(0.5*u(1)/(u(1)+u(3)))+(u(2)>0)*u(1)
  T2_pr : Fcn  Expr=(u(2)<=0)*(0.5*u(3)/(u(1)+u(3)))+(u(2)>0)*u(3)
  T_ : Fcn  Expr=0.5*(abs(u(1))-abs(u(2))/sqrt(3))
  T_1 : Fcn  Expr=abs(u(2))/sqrt(3)
  duty_A : Fcn  Expr=u(3)
  duty_B : Fcn  Expr=1-(u(3)+2*u(1))
  duty_C : Fcn  Expr=1-u(3)
  duty_ABC : Outport  OutputWhenDisabled=reset  InitialOutput=[0 0 0]
  wires:
  Mux/1 -> duty_ABC/1
  [T0] -> Mux2/3
  [T2] -> Mux2/2
  [T1] -> Mux2/1
  Mux1/1 -> T0_pr/1, T2_pr/1, T1_pr/1
  Sum/1 -> Mux1/2
  Constant/1 -> Sum/2
  vq/1 -> Mux3/2
  vd/1 -> Mux3/1
  Mux3/1 -> T_1/1, T_/1
  T_1/1 -> Mux1/1, Sum/1
  T_/1 -> Mux1/3, Sum/3
  duty_A/1 -> Mux/1
  Mux2/1 -> duty_A/1, duty_B/1, duty_C/1
  duty_B/1 -> Mux/2
  duty_C/1 -> Mux/3
  T1_pr/1 -> [T1]
  T2_pr/1 -> [T2]
  T0_pr/1 -> [T0]

== system wt_blockset_beta/Power Converters/Switching SVM Strategy/3rd quadrant/Sector 4 ==
  note: Sector 4
  vd : Inport
  vq : Inport  Port=2
  Action Port : ActionPort  InitializeStates=reset
  Constant : Constant  Value=0.5
  Mux : Mux  Inputs=3
  Mux1 : Mux  Inputs=3
  Mux2 : Mux  Inputs=3
  Mux3 : Mux  Inputs=2
  Sum : Sum  Inputs=-+-  SaturateOnIntegerOverflow=on
  T0_pr : Fcn  Expr=(u(2)<=0)*0+(u(2)>0)*u(2)
  T1_pr : Fcn  Expr=(u(2)<=0)*(0.5*u(1)/(u(1)+u(3)))+(u(2)>0)*u(1)
  T2_pr : Fcn  Expr=(u(2)<=0)*(0.5*u(3)/(u(1)+u(3)))+(u(2)>0)*u(3)
  T_1 : Fcn  Expr=0.5*(-u(1)+abs(u(2))/sqrt(3))
  T_2 : Fcn  Expr=0.5*(u(1)+abs(u(2))/sqrt(3))
  duty_A : Fcn  Expr=1-(u(3)+2*u(1))
  duty_B : Fcn  Expr=u(3)
  duty_C : Fcn  Expr=1-u(3)
  duty_ABC : Outport  OutputWhenDisabled=reset  InitialOutput=[0 0 0]
  wires:
  Sum/1 -> Mux1/2
  Constant/1 -> Sum/2
  T_1/1 -> Sum/1, Mux1/1
  T_2/1 -> Mux1/3, Sum/3
  Mux1/1 -> T1_pr/1, T2_pr/1, T0_pr/1
  [T1] -> Mux2/1
  [T2] -> Mux2/2
  [T0] -> Mux2/3
  Mux/1 -> duty_ABC/1
  Mux2/1 -> duty_A/1, duty_B/1, duty_C/1
  duty_A/1 -> Mux/1
  Mux3/1 -> T_1/1, T_2/1
  vq/1 -> Mux3/2
  vd/1 -> Mux3/1
  duty_B/1 -> Mux/2
  duty_C/1 -> Mux/3
  T1_pr/1 -> [T1]
  T2_pr/1 -> [T2]
  T0_pr/1 -> [T0]

== system wt_blockset_beta/Power Converters/Switching SVM Strategy/4th quadrant/Sector 4 ==
  note: Sector 4
  vd : Inport
  vq : Inport  Port=2
  Action Port : ActionPort  InitializeStates=reset
  Constant : Constant  Value=0.5
  Mux : Mux  Inputs=3
  Mux1 : Mux  Inputs=3
  Mux2 : Mux  Inputs=3
  Mux3 : Mux  Inputs=2
  Sum : Sum  Inputs=-+-  SaturateOnIntegerOverflow=on
  T0_pr : Fcn  Expr=(u(2)<=0)*0+(u(2)>0)*u(2)
  T1_pr : Fcn  Expr=(u(2)<=0)*(0.5*u(1)/(u(1)+u(3)))+(u(2)>0)*u(1)
  T2_pr : Fcn  Expr=(u(2)<=0)*(0.5*u(3)/(u(1)+u(3)))+(u(2)>0)*u(3)
  T_1 : Fcn  Expr=0.5*(-u(1)+abs(u(2))/sqrt(3))
  T_2 : Fcn  Expr=0.5*(u(1)+abs(u(2))/sqrt(3))
  duty_A : Fcn  Expr=1-(u(3)+2*u(1))
  duty_B : Fcn  Expr=u(3)
  duty_C : Fcn  Expr=1-u(3)
  duty_ABC : Outport  OutputWhenDisabled=reset  InitialOutput=[0 0 0]
  wires:
  duty_C/1 -> Mux/3
  duty_B/1 -> Mux/2
  vd/1 -> Mux3/1
  vq/1 -> Mux3/2
  Mux3/1 -> T_2/1, T_1/1
  duty_A/1 -> Mux/1
  Mux2/1 -> duty_C/1, duty_B/1, duty_A/1
  Mux/1 -> duty_ABC/1
  [T0] -> Mux2/3
  [T2] -> Mux2/2
  [T1] -> Mux2/1
  Mux1/1 -> T0_pr/1, T2_pr/1, T1_pr/1
  T_2/1 -> Sum/3, Mux1/3
  T_1/1 -> Mux1/1, Sum/1
  Constant/1 -> Sum/2
  Sum/1 -> Mux1/2
  T1_pr/1 -> [T1]
  T2_pr/1 -> [T2]
  T0_pr/1 -> [T0]

== system wt_blockset_beta/Power Converters/Switching SVM Strategy/4th quadrant/Sector 5 ==
  note: Sector 5
  vd : Inport
  vq : Inport  Port=2
  Action Port : ActionPort  InitializeStates=reset
  Constant : Constant  Value=0.5
  Mux : Mux  Inputs=3
  Mux1 : Mux  Inputs=3
  Mux2 : Mux  Inputs=3
  Mux3 : Mux  Inputs=2
  Sum : Sum  Inputs=-+-  SaturateOnIntegerOverflow=on
  T0_pr : Fcn  Expr=(u(2)<=0)*0+(u(2)>0)*u(2)
  T1_pr : Fcn  Expr=(u(2)<=0)*(0.5*u(1)/(u(1)+u(3)))+(u(2)>0)*u(1)
  T2_pr : Fcn  Expr=(u(2)<=0)*(0.5*u(3)/(u(1)+u(3)))+(u(2)>0)*u(3)
  T_1 : Fcn  Expr=0.5*((u(1))-abs(u(2))/sqrt(3))
  T_2 : Fcn  Expr=abs(u(2))/sqrt(3)
  duty_A : Fcn  Expr=1-u(3)
  duty_B : Fcn  Expr=u(3)
  duty_C : Fcn  Expr=1-(u(3)+2*u(1))
  duty_ABC : Outport  OutputWhenDisabled=reset  InitialOutput=[0 0 0]
  wires:
  vd/1 -> Mux3/1
  vq/1 -> Mux3/2
  Constant/1 -> Sum/2
  Sum/1 -> Mux1/2
  Mux1/1 -> T1_pr/1, T2_pr/1, T0_pr/1
  [T1] -> Mux2/1
  [T2] -> Mux2/2
  [T0] -> Mux2/3
  Mux/1 -> duty_ABC/1
  T_2/1 -> Mux1/3, Sum/3
  T_1/1 -> Mux1/1, Sum/1
  Mux3/1 -> T_1/1, T_2/1
  duty_A/1 -> Mux/1
  duty_B/1 -> Mux/2
  duty_C/1 -> Mux/3
  Mux2/1 -> duty_B/1, duty_A/1, duty_C/1
  T1_pr/1 -> [T1]
  T2_pr/1 -> [T2]
  T0_pr/1 -> [T0]

== system wt_blockset_beta/Electrical Machinery/Simulink Blocks  based Models/Salient-Pole Synchronous Machine constant parameters/Mathematical model/dq / abc ==
  D : Inport
  Q : Inport  Port=2
  theta : Inport  Port=3
  Mux : Mux  Inputs=3
  va : Fcn  Expr=u[1]*cos(u[3])-u[2]*sin(u[3])
  vb : Fcn  Expr=u[1]*cos(u[3]-2*pi/3)-u[2]*sin(u[3]-2*pi/3)
  vc : Fcn  Expr=u[1]*cos(u[3]+2*pi/3)-u[2]*sin(u[3]+2*pi/3)
  A : Outport  InitialOutput=0
  B : Outport  Port=2  InitialOutput=0
  C : Outport  Port=3  InitialOutput=0
  wires:
  va/1 -> A/1
  vb/1 -> B/1
  vc/1 -> C/1
  Mux/1 -> va/1, vb/1, vc/1
  D/1 -> Mux/1
  Q/1 -> Mux/2
  theta/1 -> Mux/3

== system wt_blockset_beta/Mechanical Components/Wind Model SB-2/3rd_Harmonic_Filter1/3rd harmonic Filter/Coefficients ==
  avg_wind : Inport
  BD coeff : Fcn  Expr=0.2766/0.3691/(r/u(1))
  CD coeff : Fcn  Expr=0.0307/0.3691/(r/u(1))^2
  ED coeff : Fcn  Expr=1.7722/0.3691/(r/u(1))
  FD coeff : Fcn  Expr=1/0.3691/(r/u(1))^2
  BD : Outport
  CD : Outport  Port=2
  ED : Outport  Port=3
  FD : Outport  Port=4
  wires:
  avg_wind/1 -> BD coeff/1, CD coeff/1, ED coeff/1, FD coeff/1
  BD coeff/1 -> BD/1
  CD coeff/1 -> CD/1
  ED coeff/1 -> ED/1
  FD coeff/1 -> FD/1

== system wt_blockset_beta/Mechanical Components/Wind Model SB-2/3rd_Harmonic_Filter2/3rd harmonic Filter/Coefficients ==
  avg_wind : Inport
  BD coeff : Fcn  Expr=0.2766/0.3691/(r/u(1))
  CD coeff : Fcn  Expr=0.0307/0.3691/(r/u(1))^2
  ED coeff : Fcn  Expr=1.7722/0.3691/(r/u(1))
  FD coeff : Fcn  Expr=1/0.3691/(r/u(1))^2
  BD : Outport
  CD : Outport  Port=2
  ED : Outport  Port=3
  FD : Outport  Port=4
  wires:
  FD coeff/1 -> FD/1
  ED coeff/1 -> ED/1
  CD coeff/1 -> CD/1
  BD coeff/1 -> BD/1
  avg_wind/1 -> FD coeff/1, ED coeff/1, CD coeff/1, BD coeff/1

== system wt_blockset_beta/Mechanical Components/Wind Model SB-2/Kaimal_Filter_1/Kaimal Filter/Coefficients ==
  avg_wind : Inport
  BD coeff : Fcn  Expr=1.3653/1.3463/(L/2/pi/u(1))
  CD coeff : Fcn  Expr=0.9846/1.3463/(L/2/pi/u(1))^2
  ED coeff : Fcn  Expr=3.7593/1.3463/(L/2/pi/u(1))
  FD coeff : Fcn  Expr=1/1.3463/(L/2/pi/u(1))^2
  BD : Outport
  CD : Outport  Port=2
  ED : Outport  Port=3
  FD : Outport  Port=4
  wires:
  avg_wind/1 -> BD coeff/1, CD coeff/1, ED coeff/1, FD coeff/1
  BD coeff/1 -> BD/1
  CD coeff/1 -> CD/1
  ED coeff/1 -> ED/1
  FD coeff/1 -> FD/1

== system wt_blockset_beta/Mechanical Components/Wind Model SB-2/Kaimal_Filter_2/Kaimal Filter/Coefficients ==
  avg_wind : Inport
  BD coeff : Fcn  Expr=1.3653/1.3463/(L/2/pi/u(1))
  CD coeff : Fcn  Expr=0.9846/1.3463/(L/2/pi/u(1))^2
  ED coeff : Fcn  Expr=3.7593/1.3463/(L/2/pi/u(1))
  FD coeff : Fcn  Expr=1/1.3463/(L/2/pi/u(1))^2
  BD : Outport
  CD : Outport  Port=2
  ED : Outport  Port=3
  FD : Outport  Port=4
  wires:
  FD coeff/1 -> FD/1
  ED coeff/1 -> ED/1
  CD coeff/1 -> CD/1
  BD coeff/1 -> BD/1
  avg_wind/1 -> FD coeff/1, ED coeff/1, CD coeff/1, BD coeff/1

== system wt_blockset_beta/Mechanical Components/Wind Model SB-2/Kaimal_Filter_3/Kaimal Filter/Coefficients ==
  avg_wind : Inport
  BD coeff : Fcn  Expr=1.3653/1.3463/(L/2/pi/u(1))
  CD coeff : Fcn  Expr=0.9846/1.3463/(L/2/pi/u(1))^2
  ED coeff : Fcn  Expr=3.7593/1.3463/(L/2/pi/u(1))
  FD coeff : Fcn  Expr=1/1.3463/(L/2/pi/u(1))^2
  BD : Outport
  CD : Outport  Port=2
  ED : Outport  Port=3
  FD : Outport  Port=4
  wires:
  avg_wind/1 -> BD coeff/1, CD coeff/1, ED coeff/1, FD coeff/1
  BD coeff/1 -> BD/1
  CD coeff/1 -> CD/1
  ED coeff/1 -> ED/1
  FD coeff/1 -> FD/1

== system wt_blockset_beta/Mechanical Components/Wind Model SB-2/ZERO_Harmonic_Filter/ZERO harmonic Filter/Coefficients ==
  avg_wind : Inport
  BD coeff : Fcn  Expr=4.7869/7.6823/(r/u(1))
  CD coeff : Fcn  Expr=0.9904/7.6823/(r/u(1))^2
  ED coeff : Fcn  Expr=7.3518/7.6823/(r/u(1))
  FD coeff : Fcn  Expr=1/7.6823/(r/u(1))^2
  BD : Outport
  CD : Outport  Port=2
  ED : Outport  Port=3
  FD : Outport  Port=4
  wires:
  FD coeff/1 -> FD/1
  ED coeff/1 -> ED/1
  CD coeff/1 -> CD/1
  BD coeff/1 -> BD/1
  avg_wind/1 -> FD coeff/1, ED coeff/1, CD coeff/1, BD coeff/1
